simulink model "FMUunsteadyBEMTs"  (R2024b)
settings: Solver=VariableStepAuto  StartTime=0.0  StopTime=10.0  RelTol=1e-3
settings Model: ExtModeTrigDuration=100  Creator=thogan1  LastModifiedBy=thogan1

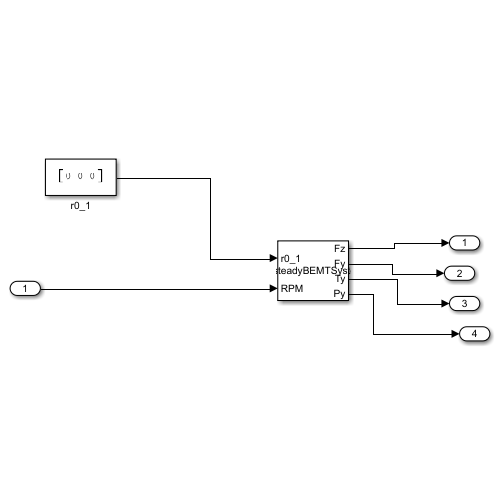
[thumbnail: Simulink's stored preview of the top-level diagram]
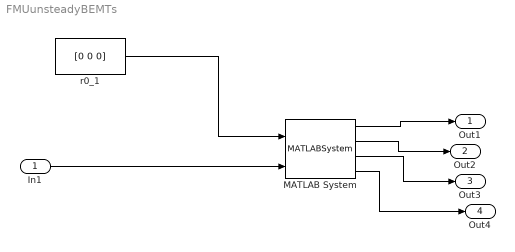
== system FMUunsteadyBEMTs ==
  In1 : Inport
  MATLAB System : MATLABSystem  System=unsteadyBEMTSystem  dt=0.01  rho=1.225  kinVisc=1.5e-5  windSpeed_nom=2  hhub_nom=25  alphaPowerLaw=1 / 5  betaBedRoughness=1  a=2  towerShadow=true  yaw=0  tilt=0  cone=5  prandtlCorrection=true  prandtlTipLoss=true  prandtlHubLoss=true  glauertCorrection=true  dynamicStall=true  dynamicWake=true  skewedWake=false  ac=1 / 3  Rr=20.5  Rh=3.5  Rb=[ 4.5, 5.5, 6.5, 7.5, 8.5, 9.5, 10.5, 11.5, 12.5, 13.5, 14.5, 15.5, 16.5, 17.5, 18.5, 19.5, 20.3 ]  chord=[ 1.63, 1.597, 1.540, 1.481, 1.420, 1.356, 1.294, 1.229, 1.163, 1.095, 1.026, 0.955, 0.881, 0.806, 0.705, 0.545, 0.265 ]  twist=[ 20.0, 16.3, 13.0, 10.05, 7.45, 5.85, 4.85, 4.00, 3.15, 2.60, 2.02, 1.36, 0.77, 0.33, 0.14, 0.05, 0.02 ]  pitch=0.01  nB=3  n=[ 0, 0, -1 ]  linThresh=0.85  polarData=load( 'polarData.mat', 'polarData' )  nDoF=3  SimulateUsing=Code generation
      mask Type: unsteadyBEMTSystem
      mask Display:
      | disp('unsteadyBEMTSystem');
      | port_label('input',1,'r0_1');
      | port_label('input',2,'RPM');
      | port_label('output',1,'Fz');
      | port_label('output',2,'Fy');
      | port_label('output',3,'Ty');
      | port_label('output',4,'Py');
  r0_1 : Constant  Value=[0 0 0]
  Out1 : Outport
  Out2 : Outport  Port=2
  Out3 : Outport  Port=3
  Out4 : Outport  Port=4
  wires:
  r0_1/1 -> MATLAB System/1
  In1/1 -> MATLAB System/2
  MATLAB System/1 -> Out1/1
  MATLAB System/2 -> Out2/1
  MATLAB System/3 -> Out3/1
  MATLAB System/4 -> Out4/1
